simulink model "general_mod"  (Simulink 3.00)
settings: Solver=ode45  StartTime=0.0  StopTime=100.0  RelTol=1e-3
values from neighbouring files (symbols this model uses):
  stack = struct('general',[],'evaluation',[],'simulation',[],'temp',[])    [gohome.m]
settings Model: SaveTime=off  SaveOutput=off

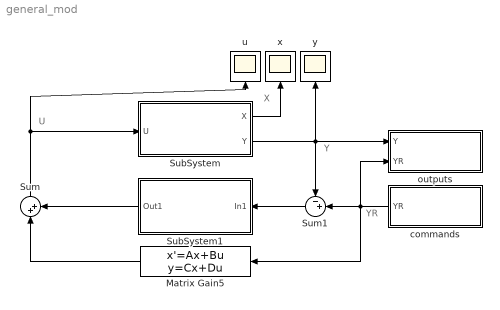
== system general_mod ==
  note: U
  note: Y
  note: YR
  note: X
  Matrix Gain5 : StateSpace  Orientation=left  A=[]  B=[]  C=[]  D=stack.simulation.pinvG0  X0=0
      mask Display: disp('pinv( G( 0 ) )')
  SubSystem : Subsystem
      mask Display: disp('PLANT')
  SubSystem1 : Subsystem  Orientation=left
      mask Display: disp('CONTROLLER')
  Sum : Sum  Orientation=up  Inputs=|++  SaturateOnIntegerOverflow=on
  Sum1 : Sum  Orientation=left  Inputs=-+|  SaturateOnIntegerOverflow=on
  commands : Subsystem  Orientation=left
      mask Display: disp('COMMANDS')
  outputs : Subsystem
      mask Display: disp('OUTPUTS')
  u : Scope
      settings: Orientation=up  TimeRange=auto  YMin=-5  YMax=5  SaveToWorkspace=off  SaveName=ScopeData
  x : Scope
      settings: Orientation=up  TimeRange=auto  YMin=-5  YMax=5  SaveToWorkspace=off  SaveName=ScopeData
  y : Scope
      settings: Orientation=up  TimeRange=auto  YMin=-5  YMax=5  SaveToWorkspace=off  SaveName=ScopeData
  wires:
  SubSystem1/1(Out1) -> Sum/2
  Matrix Gain5/1 -> Sum/1
  Sum1/1 -> SubSystem1/1(In1)
  SubSystem/1(X) -> x/1
  Sum/1 -> SubSystem/1(U), u/1
  SubSystem/2(Y) -> outputs/1(Y), y/1, Sum1/1
  commands/1(YR) -> Matrix Gain5/1, outputs/2(YR), Sum1/2

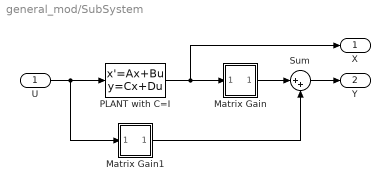
== system general_mod/SubSystem ==
  U : Inport  Port=1  PortWidth=-1  SampleTime=-1  DataType=auto
      settings: SignalType=auto
  Matrix Gain : Subsystem  mask(Matrix Gain){K=stack.general.C}
      mask prompts: K "Gain matrix:"
      mask help: Matrix Gain.
      mask Help: Multiplies input vector by entered matrix to produce output vector (y=Au).
      mask Display: disp('C')
  Matrix Gain1 : Subsystem  mask(Matrix Gain){K=stack.general.D}
      mask prompts: K "Gain matrix:"
      mask help: Matrix Gain.
      mask Help: Multiplies input vector by entered matrix to produce output vector (y=Au).
      mask Display: disp('D')
  PLANT with C=I : StateSpace  A=stack.general.A  B=stack.general.B  C=eye(size(stack.general.A))  D=zeros(size(stack.general.A,1),size(stack.general.B,2))  X0=0
  Sum : Sum  Inputs=|++  SaturateOnIntegerOverflow=on
  X : Outport  Port=1
  Y : Outport  Port=2
  wires:
  Matrix Gain/1(Out1) -> Sum/1
  Sum/1 -> Y/1
  PLANT with C=I/1 -> Matrix Gain/1(In1), X/1
  Matrix Gain1/1(Out1) -> Sum/2
  U/1 -> PLANT with C=I/1, Matrix Gain1/1(In1)

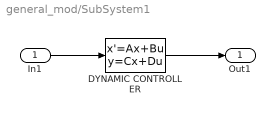
== system general_mod/SubSystem1 ==
  In1 : Inport  Port=1  PortWidth=-1  SampleTime=-1  DataType=auto
      settings: SignalType=auto
  DYNAMIC CONTROLLER : StateSpace  A=stack.simulation.Ak  B=stack.simulation.Bk  C=stack.simulation.Ck  D=stack.simulation.Dk  X0=0
  Out1 : Outport  Port=1
  wires:
  In1/1 -> DYNAMIC CONTROLLER/1
  DYNAMIC CONTROLLER/1 -> Out1/1

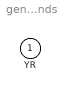
== system general_mod/commands ==
  YR : Outport  Orientation=left  Port=1

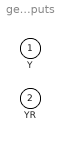
== system general_mod/outputs ==
  Y : Inport  Port=1  PortWidth=-1  SampleTime=-1  DataType=auto
      settings: SignalType=auto
  YR : Inport  Port=2  PortWidth=-1  SampleTime=-1  DataType=auto
      settings: SignalType=auto

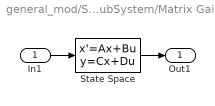
== system general_mod/SubSystem/Matrix Gain ==
  In1 : Inport  Port=1  PortWidth=-1  SampleTime=-1  DataType=auto
      settings: SignalType=auto
  State Space : StateSpace  A=[]  B=[]  C=[]  D=K  X0=0
  Out1 : Outport  Port=1
  wires:
  In1/1 -> State Space/1
  State Space/1 -> Out1/1

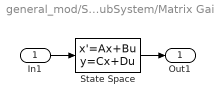
== system general_mod/SubSystem/Matrix Gain1 ==
  In1 : Inport  Port=1  PortWidth=-1  SampleTime=-1  DataType=auto
      settings: SignalType=auto
  State Space : StateSpace  A=[]  B=[]  C=[]  D=K  X0=0
  Out1 : Outport  Port=1
  wires:
  In1/1 -> State Space/1
  State Space/1 -> Out1/1
